simulink model "sl_groundvehicleDynamics_AP"  (R2025a)
settings: Solver=ode45  StartTime=0.0  StopTime=2000  RelTol=1e-5  EnableMultiTasking=on
InitFcn:
  | mdl_robot;
undefined symbols (not defined in the file): Ordered_Waypoints, robot
libraries: simulink x4, mobileRoboticsLib x3, simulink_extras x2
settings Model: Creator=sriramn  LastModifiedBy=hunte
settings SolverCC: ZeroCrossAlgorithm=Adaptive  AlgebraicLoopSolver=TrustRegion
settings DataIOCC: LimitDataPoints=on  SaveFormat=Array  ReturnWorkspaceOutputs=off
settings OptimizationCC: ReuseModelBlockBuffer=off  LifeSpan=inf
settings DebuggingCC: SolverPrmCheckMsg=warning  UnconnectedInputMsg=warning  UnconnectedOutputMsg=warning  UnconnectedLineMsg=warning  AllowSymbolicDim=off  SFUnexpectedBacktrackingDiag=warning  SFNoUnconditionalDefaultTransitionDiag=warning  SFExecutionAtInitializationDiag=none  UnderSpecifiedDimensionMsg=warning  ArithmeticOperatorsInVariantConditions=warning
settings HardwareCC: ProdBitPerPointer=32.0  ProdBitPerSizeT=32.0  ProdBitPerPtrDiffT=32.0  ProdLargestAtomicFloat=None  ProdIntDivRoundTo=Undefined  ProdEndianess=Unspecified  ProdWordSize=32.0  ProdHWDeviceType=32-bit Generic
settings ModelReferenceCC: EnableRefExpFcnMdlSchedulingChecks=on  ModelReferenceMinAlgLoopOccurrences=on  PropagateSignalLabelsOutOfModel=off
settings SFSimCC: SimUseLocalCustomCode=off  CustomCodeUndefinedFunction=UseInterfaceOnly
settings RTWCC: RTWUseLocalCustomCode=off  GPUComputeCapability=3.5
settings CodeAppCC: StateflowObjectComments=on
settings GRTTargetCC: TargetLangStandard=C89/C90 (ANSI)
settings ConfigComp: CovMetricSettings=dw  CovSaveCumulativeToWorkspaceVar=on  CovSaveSingleToWorkspaceVar=on  CovExternalEMLEnable=off  CovSFcnEnable=off
settings SimscapeCC: SimscapeNormalizeSystem=off
settings ConfigurationSet: Description=SimMechanics 2G
settings ExplorerConfigSet: InternalSimMechanicsExplorerSettings="<ExplorerConfiguration><canonicalview>planar_xy</canonicalview><AnimationSetting><BasePlaybackSpeed>1.0</BasePlaybackSpeed><PlaybackSpeedFactor>1.0</PlaybackSpeedFactor></AnimationSetting><TilePanel><TileInfo><Tiles Columns=\"1\" Count=\"1\" Rows=\"1\"><Column Left=\"2\" Weight=\"1\"/><Column Left=\"1628\"/><Row Top=\"2\" Weight=\"1\"/><Row Top=\"1072\"/><Tile Height=\"1\" Width=\"1\" X=\"0\" Y=\"0\"/></Tiles></TileInfo><SceneInfo><SceneViewer><BGColor><R>0.60000002384185791</R><G>0.60000002384185791</G><B>0.60000002384185791</B></BGColor><Camera><Position><X>0.22951840878551699</X><Y>0.32651610611526627</Y><Z>-0.27215421354393321</Z></Position><Center><X>-0.15775714411666431</X><Y>-0.15462825985839526</Y><Z>0.065702552916005602</Z></Center><Up><X>-0.56030137557930915</X><Y>0.72817587161684794</Y><Z>0.39474329445726858</Z></Up><Left>-0.21481383955700509</Left><Right>0.21481383955700509</Right><Bottom>-0.27569784609469139</Bottom><Top>0.27569784609469139</Top></Camera></SceneViewer></SceneInfo></TilePanel></ExplorerConfiguration>"

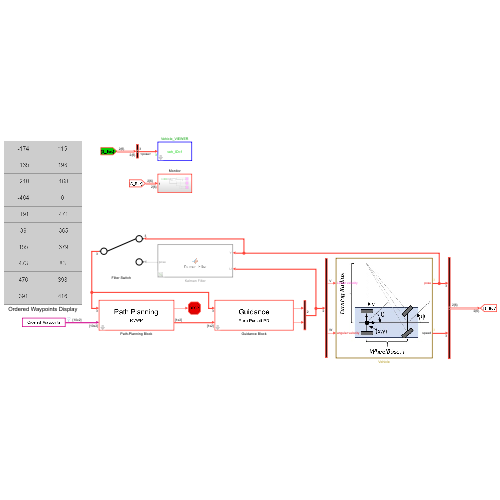
[thumbnail: Simulink's stored preview of the top-level diagram]
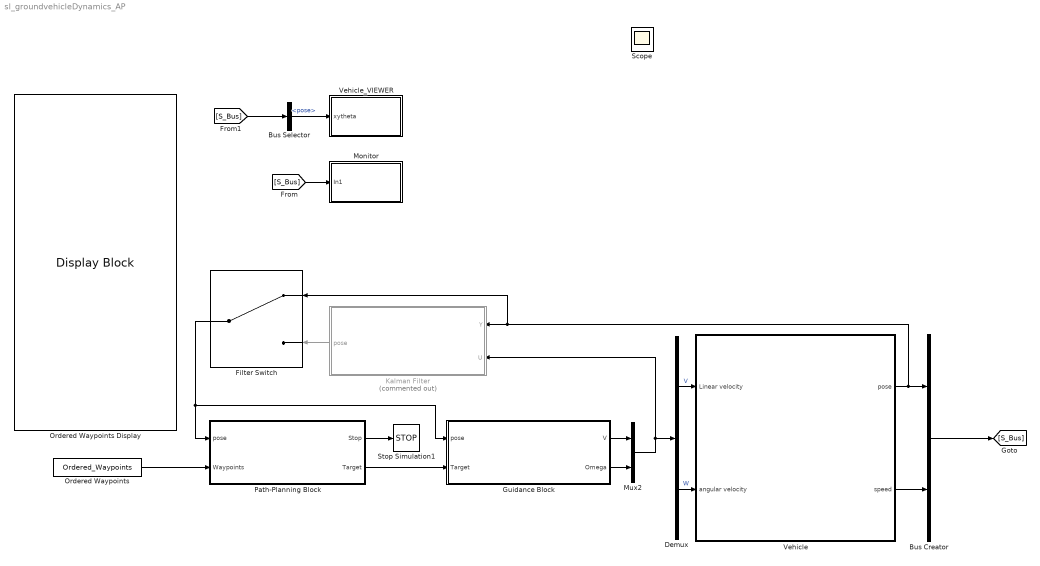
== system sl_groundvehicleDynamics_AP ==
  Bus Creator : BusCreator  Inputs=2
  Bus Selector : BusSelector  OutputSignals=pose
  Demux : Demux  Outputs=2
  Filter Switch : ManualSwitch
  Guidance Block : MATLAB Function  TreatAsAtomicUnit=on  mask{Vc=150, Kp=10, Kd=1, N=4}
      mask prompts: Vc "Linear Velocity [V]:"; Kp "Proportional Gain [Kp]:"; Kd "Derivative Gain [Kd]:"; N "Navigation Gain [N]:"
  Kalman Filter : MATLAB Function  Commented=on  TreatAsAtomicUnit=on
  Monitor : Subsystem
  Mux2 : Mux  Inputs=2
  Ordered Waypoints : Constant  Value=Ordered_Waypoints  VectorParams1D=off
  Ordered Waypoints Display : DisplayBlock  LabelPosition=Hide  Transparency=1  GridColor=[0.502, 0.502, 0.502]
  Path-Planning Block : MATLAB Function  TreatAsAtomicUnit=on  mask{Init_Pos=[0, 0], LookAhead=2, WP_Thresh=6}
      mask prompts: Init_Pos "Initial Position [X0, Y0]:"; LookAhead "Look-Ahead Distance [Ahead]:"; WP_Thresh "WayPoint Threshold [WP_Thresh]:"
  Stop Simulation1 : Stop
  Vehicle : Subsystem
      mask Display: image('vehicle.jpg');
  Vehicle_VIEWER : Subsystem  mask{wp_mat=[-500, 500; -500, 500]', veh_ID_num=1, veh_init_xytheta=[robot.X robot.Y robot.Theta], Ts=0.5}
      mask prompts: wp_mat "Waypoint matrix for arena [x_col, y_col] (m)"; veh_ID_num "Vehicle ID number"; veh_init_xytheta "Initial pose [x,y,theta]"; Ts "Sample time for updating animation (secs)"
      mask TypeOptions veh_ID_num: 1 | 2 | 3 | 4
      mask DialogControl Control2 Prompt: Animate simulation of Differential Drive Robot (DDR)
      mask Display: fprintf('veh_ID=%d',veh_ID_num);
  Scope : Scope
      settings: ActiveDisplayYMinimum=0.07  ActiveDisplayYMaximum=0.09
  wires:
  [S_Bus] -> Monitor/1(In1)
  [S_Bus] -> Bus Selector/1
  Vehicle/2(speed) -> Bus Creator/2
  Bus Creator/1 -> [S_Bus]
  Bus Selector/1 -> Vehicle_VIEWER/1(xytheta)  "<pose>"
  Filter Switch/1 -> Guidance Block/1(pose), Path-Planning Block/1(pose)
  Demux/1 -> Vehicle/1(Linear velocity)  "V"
  Guidance Block/2(Omega) -> Mux2/2
  Guidance Block/1(V) -> Mux2/1
  Demux/2 -> Vehicle/2(angular velocity)  "W"
  Mux2/1 -> Kalman Filter/2(U), Demux/1
  Path-Planning Block/2(Target) -> Guidance Block/2(Target)
  Ordered Waypoints/1 -> Path-Planning Block/2(Waypoints)
  Vehicle/1(pose) -> Bus Creator/1, Filter Switch/1, Kalman Filter/1(Y)
  Path-Planning Block/1(Stop) -> Stop Simulation1/1
  Kalman Filter/1(pose) -> Filter Switch/2

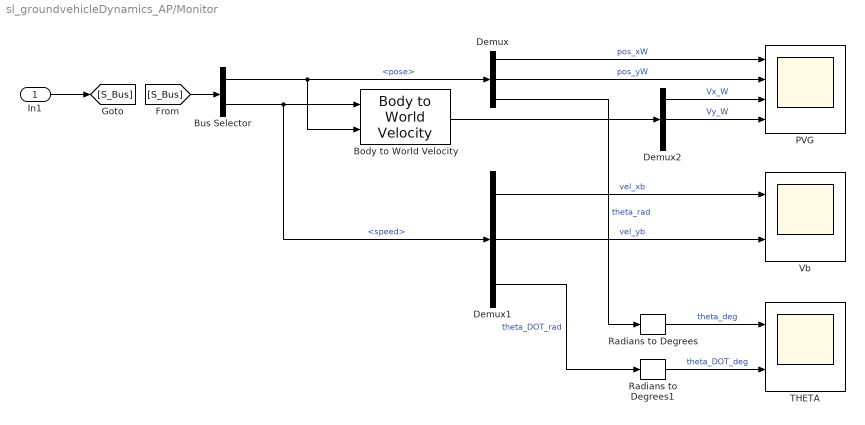
== system sl_groundvehicleDynamics_AP/Monitor ==
  In1 : Inport
  Body to World Velocity : mobileRoboticsLib/Utilities/Body to World Velocity
      settings: SourceProductName=Mobile Robotics Simulation Toolbox
  Bus Selector : BusSelector  OutputSignals=pose,speed
  Demux : Demux  Outputs=3
  Demux1 : Demux  Outputs=3
  Demux2 : Demux  Outputs=3
  PVG : Scope  NumInputPorts=4
      settings: ActiveDisplayYMinimum=-3.02358  ActiveDisplayYMaximum=27.35477
  Radians to Degrees : simulink_extras/Transformations/Radians to Degrees
  Radians to Degrees1 : simulink_extras/Transformations/Radians to Degrees
  THETA : Scope  NumInputPorts=2
      settings: ActiveDisplayYMinimum=-8.72937  ActiveDisplayYMaximum=60.06611  DataLoggingVariableName=ScopeData2
  Vb : Scope  NumInputPorts=2
      settings: ActiveDisplayYMinimum=0.05577  ActiveDisplayYMaximum=0.8929
  wires:
  In1/1 -> [S_Bus]
  [S_Bus] -> Bus Selector/1
  Demux/1 -> PVG/1  "pos_xW"
  Demux/2 -> PVG/2  "pos_yW"
  Radians to Degrees1/1 -> THETA/2  "theta_DOT_deg"
  Radians to Degrees/1 -> THETA/1  "theta_deg"
  Demux1/3 -> Radians to Degrees1/1  "theta_DOT_rad"
  Demux/3 -> Radians to Degrees/1  "theta_rad"
  Bus Selector/1 -> Body to World Velocity/2, Demux/1  "<pose>"
  Bus Selector/2 -> Demux1/1, Body to World Velocity/1  "<speed>"
  Body to World Velocity/1 -> Demux2/1
  Demux2/1 -> PVG/3  "Vx_W"
  Demux2/2 -> PVG/4  "Vy_W"
  Demux1/1 -> Vb/1  "vel_xb"
  Demux1/2 -> Vb/2  "vel_yb"

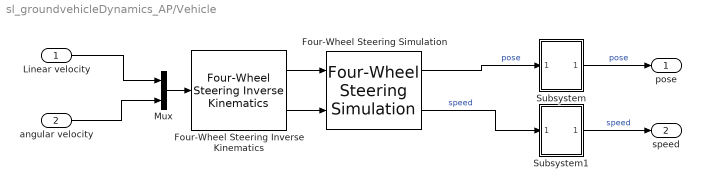
== system sl_groundvehicleDynamics_AP/Vehicle ==
  Linear velocity : Inport
  angular velocity : Inport  Port=2
  Four-Wheel Steering Inverse Kinematics : mobileRoboticsLib/Kinematic Models/Four-Wheel Steering/Four-Wheel Steering Inverse Kinematics  wheelRadius=0.1  frontWheelDist=0.25  rearWheelDist=0.25  ikMode=Front Steering
      settings: SourceProductName=Mobile Robotics Simulation Toolbox
  Four-Wheel Steering Simulation : mobileRoboticsLib/Kinematic Models/Four-Wheel Steering/Four-Wheel Steering Simulation  wheelRadius=0.1  frontWheelDist=0.25  rearWheelDist=0.25  initX=robot.X  initY=robot.Y  initAngle=robot.Theta  Ts=0.05
      settings: SourceProductName=Mobile Robotics Simulation Toolbox
  Mux : Mux  Inputs=2
  Subsystem : Subsystem
  Subsystem1 : Subsystem
  pose : Outport  VectorParamsAs1DForOutWhenUnconnected=off
  speed : Outport  Port=2
  wires:
  angular velocity/1 -> Mux/2
  Linear velocity/1 -> Mux/1
  Mux/1 -> Four-Wheel Steering Inverse Kinematics/1
  Four-Wheel Steering Simulation/1 -> Subsystem/1(In1)  "pose"
  Four-Wheel Steering Simulation/2 -> Subsystem1/1(In1)  "speed"
  Four-Wheel Steering Inverse Kinematics/1 -> Four-Wheel Steering Simulation/1
  Four-Wheel Steering Inverse Kinematics/2 -> Four-Wheel Steering Simulation/2
  Subsystem/1(pose) -> pose/1  "pose"
  Subsystem1/1(speed) -> speed/1  "speed"

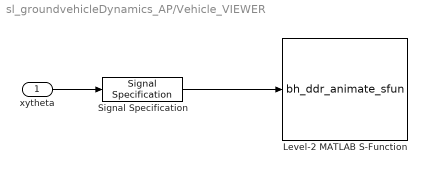
== system sl_groundvehicleDynamics_AP/Vehicle_VIEWER ==
  xytheta : Inport
  Level-2 MATLAB S-Function : M-S-Function  FunctionName=bh_ddr_animate_sfun  Parameters=Ts, Ordered_Waypoints, veh_ID_num, veh_init_xytheta
  Signal Specification : SignalSpecification  Dimensions=3
  wires:
  xytheta/1 -> Signal Specification/1
  Signal Specification/1 -> Level-2 MATLAB S-Function/1

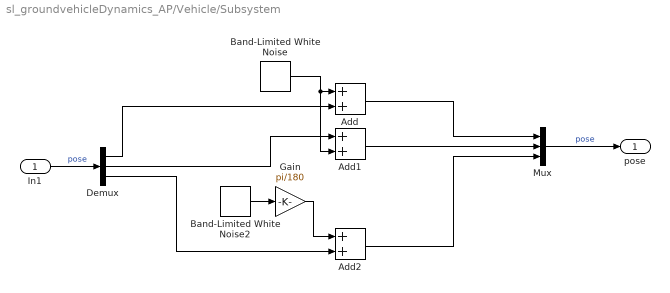
== system sl_groundvehicleDynamics_AP/Vehicle/Subsystem ==
  In1 : Inport
  Add : Sum
  Add1 : Sum
  Add2 : Sum
  Band-Limited White Noise : simulink/Sources/Band-Limited White Noise  Cov=[0.001]  Ts=0.1  seed=[23341]
  Band-Limited White Noise2 : simulink/Sources/Band-Limited White Noise  Cov=[0.41]  Ts=0.1  seed=[23341]
  Demux : Demux  Outputs=3
  Gain : Gain  Gain=pi/180
  Mux : Mux  Inputs=3
  pose : Outport
  wires:
  Add1/1 -> Mux/2
  Add2/1 -> Mux/3
  Demux/2 -> Add1/1
  Band-Limited White Noise2/1 -> Gain/1
  Demux/3 -> Add2/2
  Band-Limited White Noise/1 -> Add1/2, Add/1
  In1/1 -> Demux/1  "pose"
  Demux/1 -> Add/2
  Gain/1 -> Add2/1
  Mux/1 -> pose/1  "pose"
  Add/1 -> Mux/1

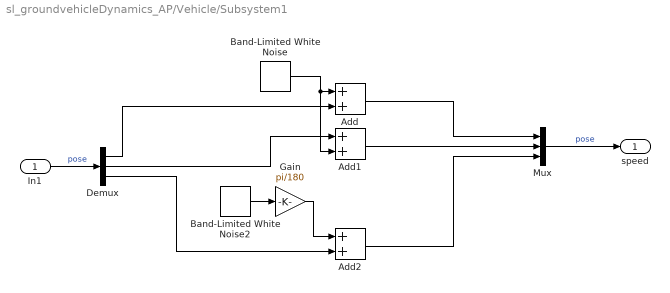
== system sl_groundvehicleDynamics_AP/Vehicle/Subsystem1 ==
  In1 : Inport
  Add : Sum
  Add1 : Sum
  Add2 : Sum
  Band-Limited White Noise : simulink/Sources/Band-Limited White Noise  Cov=[0.001]  Ts=0.1  seed=[23341]
  Band-Limited White Noise2 : simulink/Sources/Band-Limited White Noise  Cov=[0.41]  Ts=0.1  seed=[23341]
  Demux : Demux  Outputs=3
  Gain : Gain  Gain=pi/180
  Mux : Mux  Inputs=3
  speed : Outport
  wires:
  Add1/1 -> Mux/2
  Add2/1 -> Mux/3
  Demux/2 -> Add1/1
  Band-Limited White Noise2/1 -> Gain/1
  Demux/3 -> Add2/2
  Band-Limited White Noise/1 -> Add1/2, Add/1
  In1/1 -> Demux/1  "pose"
  Demux/1 -> Add/2
  Gain/1 -> Add2/1
  Mux/1 -> speed/1  "pose"
  Add/1 -> Mux/1

== matlab function sl_groundvehicleDynamics_AP/Path-Planning Block ==
  data: Stop output; Target output; pose input; Waypoints input; WP_Thresh parameter; LookAhead parameter; Init_Pos parameter
function [Stop, Target] = Path_Planning(pose, Waypoints, WP_Thresh, LookAhead, Init_Pos)


persistent WP_List;
persistent N_WPs;
persistent Target_WP_Idx;


Stop = 0;


%% Configs:

% % Distance from WP that Counts as Visited:
% WP_Thresh = 10;
% 
% % How Far Forward the RVWP should be from the Robot's Projected Position:
% LookAhead = 30;


% X-Y Position of the Robot:
Pos = [pose(1), pose(2)];


%% Parsing and Initialisation of Waypoints:

if isempty(WP_List)

    N_WPs = size(Waypoints, 1);

    WP_List = repmat(struct("Pos", zeros(1, 2), "Visited", false, "Vect", zeros(1, 2), "Len", 0, "Dir", zeros(1, 2)), 1, N_WPs);

    % Turning the List of WPs into a Struct Array:
    for k = 1:N_WPs

        WP_List(k).Pos = Waypoints(k, :);

        if k ~= 1,  WP_List(k).Vect = Waypoints(k, :) - Waypoints(k-1, :);
        else,       WP_List(k).Vect = Waypoints(k, :) - Init_Pos;
        end

        WP_List(k).Len = norm(WP_List(k).Vect);
        WP_List(k).Dir = WP_List(k).Vect / WP_List(k).Len;
    
    end

    Target_WP_Idx = 1;
end


%% Indexing Target WP:

if sqrt( (WP_List(Target_WP_Idx).Pos(1)-pose(1))^2 + (WP_List(Target_WP_Idx).Pos(2)-pose(2))^2 ) < WP_Thresh

    WP_List(Target_WP_Idx).Visited = true;

    if (Target_WP_Idx == N_WPs), Stop = 1;
    else, Target_WP_Idx = Target_WP_Idx + 1;
    end

end


%% Calculating Vector Projection onto Segment + LookAhead:


Dot_Product_Proj =  dot(WP_List(Target_WP_Idx).Dir, (Pos - WP_List(Target_WP_Idx).Pos));

Target = WP_List(Target_WP_Idx).Pos + (min((Dot_Product_Proj + LookAhead), WP_List(Target_WP_Idx).Len) * WP_List(Target_WP_Idx).Dir);

== matlab function sl_groundvehicleDynamics_AP/Kalman Filter ==
  data: Y input; U input size=2; pose output
function pose = Kalman_Filter(Y, U)

%{

Measurement     [Y]     =   [Xpos; Ypos; Theta]
Command Output  [U]     =   [V; W]

%}


%% Configs:

dt          = 0.05;                 % Sample Time.                          (known)

sig2_V      = 0.10;                 % Linear-Velocity Q-Var.                (unknown)
sig2_W      = 0.05;                 % Angular-Velocity Q-Var.               (unknown)

sig2_Xpos   = 0.01;                 % Xpos R-Var.                           (known)
sig2_Ypos   = 0.01;                 % Ypos R-Var.                           (known)
sig2_Theta  = 2*(pi/180);           % Theta R-Var.                          (known)

P0_pos      = 10^2;                 % Initial Pos Co-Var.                   (unknown)
P0_theta    = (15*pi/180)^2;        % Initial Theta Co-Var.                 (unknown)


Q   = diag([sig2_V, sig2_W]);                       % Command Variance (Q-Var).
R   = diag([sig2_Xpos, sig2_Ypos, sig2_Theta]);     % Measurement Variance (R-Var).

H   = eye(3);


%% Model State:

persistent X P
if isempty(X)
    X   = zeros(3, 1, 'like', U);
    P   = diag([P0_pos, P0_pos, P0_theta]);
end


%% Prediction:

V   = U(1);
W   = U(2);


% X_ = X + [  dt*V*cos(X(3))
%             dt*V*sin(X(3))
%             dt*W            ];

% X-bar:
X_ = X + dt*[V*cos(X(3)), V*sin(X(3)), W].';
X_(3) = wrapToPi(X_(3));


% Measurement Jacobian [F]:
F = [   1,      0,      -dt*V*sin(X(3))
        0,      1,      dt*V*cos(X(3))
        0,      0,      1               ];

% Command Jacobian [G]:
G = [ dt*cos(X(3)),     0;
      dt*sin(X(3)),     0;
      0,                dt ];

% Co-Variance [P]:
P_ = F*P*F.' + G*Q*G.';


%% Measurement:

innov       = Y(:) - X_;
innov(3)    = wrapToPi(innov(3));      % Wrap Theta residual to [-pi, pi] to avoid jumps.

% Kalman Gain [K]:
K = P_*H.'/(H*P_*H.' + R);

X = X_ + K*(innov);
X(3) = wrapToPi(X(3));

I3 = eye(3, class(U));
P = (I3 - K*H)*P_;


%% Output:

pose = X.';   % row vector [1x3] to match your bus


end

== matlab function sl_groundvehicleDynamics_AP/Guidance Block ==
  data: V output; pose input; Omega output; Target input; Vc parameter; Kp parameter; Kd parameter; N parameter
function [V, Omega] = Guidance(pose, Target, Vc, Kp, Kd, N)

persistent Last_Delta;
persistent Last_RTP;


%% Configs:

    
% V   = 1.5;      % Constant Velocity (V),    (Originally [v = 0.99])
% Kp  = 0.8;      % Proportional Gain (Kp),   (Originally [0.8])
% Kd  = 1.0;      % Derivative Gain   (Kd),   (Originally [0.8])
% N   = 4.0;      % Navigation Gain   (N),    (Ideally [3<=N<=5])


V = Vc;


%% Range and Heading:

% Flight Path Angle [Gamma], (rad):
Gamma = pose(3);


% Relative Target Position [RTP] in the inertial frame, (m):
RTP = [(Target(1) - pose(1));... % dx
    (Target(2) - pose(2))];      % dy

% Range to Target [Range], (m):
Range = norm(RTP);

% Line-Of-Sight [Lambda] Angle, (rad):
Lambda = atan2(RTP(2),RTP(1));


%% Proportional [P] (Pure Pursuite):

% Heading Error [Delta], (rad):
Delta = Lambda - Gamma;
if      (Delta < -pi),  Delta = Delta + 2*pi;
elseif  (Delta > +pi),  Delta = Delta - 2*pi;
end


%% Derivitive [D] (Proportional Navigation):

t_step = 0.1;

if isempty(Last_Delta), Last_Delta  = Delta;   end
if isempty(Last_RTP),   Last_RTP    = RTP;     end

Delta_dot   = (Delta - Last_Delta) ./ t_step;                               % Delta_dot     - Heading Error Time Derivitive.
RTP_dot     = (RTP - Last_RTP) ./ t_step;                                   % RTP_dot       - Relative Target Position Time Derivitive.
Range_dot   = norm(RTP_dot);                                                % Range_dot     - Distance to Target Time Derivitive
Lambda_dot  = ( (RTP(1)*RTP_dot(2)) - (RTP(2)*RTP_dot(1)) ) / ( Range^2 );  % Lambda_dot    - LOS Angle Time Derivitive.

Last_Delta = Delta;
Last_RTP = RTP;



%% Controller Types:

% if (abs(Delta) > pi/3)
%     if (0)
%     Omega = (Kp * Delta);                                                   % [P] Controller (Pure Pursuit).
%     else
%     Omega = (Kp * Delta) + (Kd * Delta_dot);                                % [PD] Controller (Pure Pursuit).
%     end
% else
%     Omega = (N * Lambda_dot);                                               % [D] Controller (Proportional Navigation).
% end



%% Pure Pursuit:

Omega = (Kp * Delta) + (Kd * Delta_dot);                                    % [PD] Controller (Pure Pursuit).



%% Output Logging:

% LOS         = Lambda    * (180/pi);
% Heading     = Gamma     * (180/pi);
% Lead_Angle  = Delta     * (180/pi);
% 
% LoggingOutput = [LOS Heading Lead_Angle];
